simulink model "lstm_turboShaftEngine_Harness1"  (R2024a)
settings: Solver=VariableStepAuto  StartTime=0.0  StopTime=10.0  RelTol=1e-3
settings Model: Creator=imyrsini  LastModifiedBy=imyrsini
settings RTWCC: GPUComputeCapability=3.5

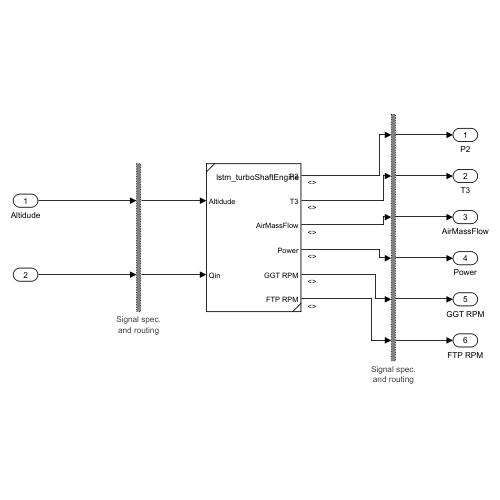
[thumbnail: Simulink's stored preview of the top-level diagram]
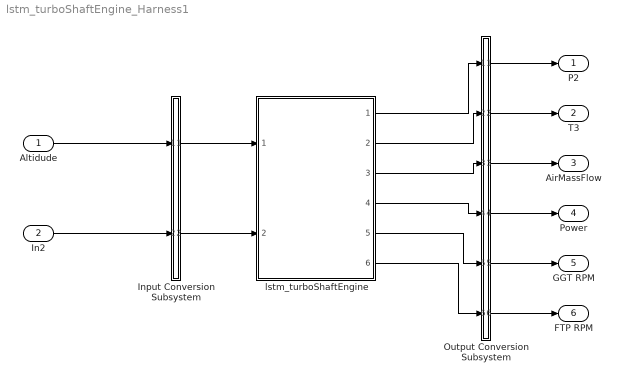
== system lstm_turboShaftEngine_Harness1 ==
  Altidude : Inport
  In2 : Inport  Port=2
  Input Conversion Subsystem : Subsystem  Tag=__SLT_ICS__  Description=|
      | Signal spec.
      | and routing
      settings: AttributesFormatString=%<Description>
  Output Conversion Subsystem : Subsystem  Tag=__SLT_OCS__  Description=|
      | Signal spec.
      | and routing
      settings: AttributesFormatString=%<Description>
  lstm_turboShaftEngine : Subsystem  ReferencedSubsystem=lstm_turboShaftEngine
  P2 : Outport
  T3 : Outport  Port=2
  AirMassFlow : Outport  Port=3
  Power : Outport  Port=4
  GGT RPM : Outport  Port=5
  FTP RPM : Outport  Port=6
  wires:
  Altidude/1 -> Input Conversion Subsystem/1(Inport_1)
  In2/1 -> Input Conversion Subsystem/2(Inport_2)
  Output Conversion Subsystem/1(Outport_1) -> P2/1
  Output Conversion Subsystem/2(Outport_2) -> T3/1
  Output Conversion Subsystem/3(Outport_3) -> AirMassFlow/1
  Output Conversion Subsystem/4(Outport_4) -> Power/1
  Output Conversion Subsystem/5(Outport_5) -> GGT RPM/1
  Output Conversion Subsystem/6(Outport_6) -> FTP RPM/1
  Input Conversion Subsystem/1(Outport_1) -> lstm_turboShaftEngine/1
  Input Conversion Subsystem/2(Outport_2) -> lstm_turboShaftEngine/2
  lstm_turboShaftEngine/1 -> Output Conversion Subsystem/1(Inport_1)
  lstm_turboShaftEngine/2 -> Output Conversion Subsystem/2(Inport_2)
  lstm_turboShaftEngine/3 -> Output Conversion Subsystem/3(Inport_3)
  lstm_turboShaftEngine/4 -> Output Conversion Subsystem/4(Inport_4)
  lstm_turboShaftEngine/5 -> Output Conversion Subsystem/5(Inport_5)
  lstm_turboShaftEngine/6 -> Output Conversion Subsystem/6(Inport_6)

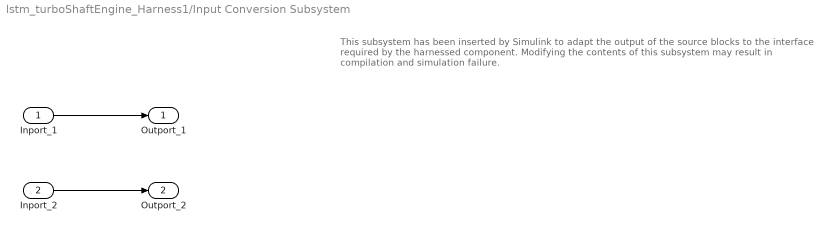
== system lstm_turboShaftEngine_Harness1/Input Conversion Subsystem ==
  note: This subsystem has been inserted by Simulink to adapt the output of the source blocks to the interface required by the harnessed component.
      |  Modifying the contents of this subsystem may result in compilation and simulation failure.
  Inport_1 : Inport
  Inport_2 : Inport  Port=2
  Outport_1 : Outport
  Outport_2 : Outport  Port=2
  wires:
  Inport_1/1 -> Outport_1/1
  Inport_2/1 -> Outport_2/1

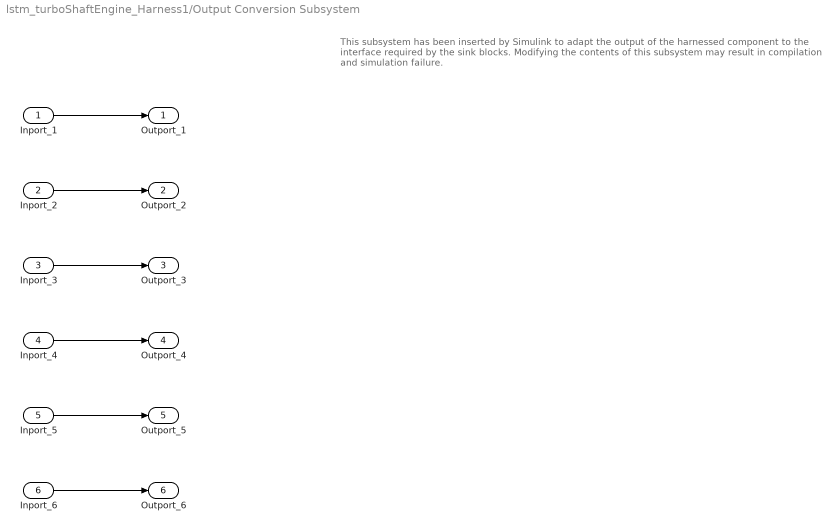
== system lstm_turboShaftEngine_Harness1/Output Conversion Subsystem ==
  note: This subsystem has been inserted by Simulink to adapt the output of the harnessed component to the interface required by the sink blocks.
      |  Modifying the contents of this subsystem may result in compilation and simulation failure.
  Inport_1 : Inport
  Inport_2 : Inport  Port=2
  Inport_3 : Inport  Port=3
  Inport_4 : Inport  Port=4
  Inport_5 : Inport  Port=5
  Inport_6 : Inport  Port=6
  Outport_1 : Outport
  Outport_2 : Outport  Port=2
  Outport_3 : Outport  Port=3
  Outport_4 : Outport  Port=4
  Outport_5 : Outport  Port=5
  Outport_6 : Outport  Port=6
  wires:
  Inport_1/1 -> Outport_1/1
  Inport_2/1 -> Outport_2/1
  Inport_3/1 -> Outport_3/1
  Inport_4/1 -> Outport_4/1
  Inport_5/1 -> Outport_5/1
  Inport_6/1 -> Outport_6/1
